simulink model "DYN_02x"  (R2021a)
settings: Solver=FixedStepAuto  StartTime=0.0  StopTime=10  FixedStep=0.01  RelTol=1e-3
(part 14 of 14)

== matlab function DYN_02x/Data ==
  data: m output; L output; Pic output; I output
function [m,L,Pic,I] = DATA_6DOF()
a1=0.75; a2=2.70; a3=0.90; d1=3.35; d4=2.95; d7=0.80;
m0 = 7.2407; m1 = 5.6511; m2 = 4.6061; m3 = 4.2963; m4 = 1.9151; m5 = 0.3399; m6 = 0.0714;
m = [m1 m2 m3 m4 m5 m6];
L = [a1 a2 a3 d1 d4 d7];
Pic = zeros(6,3);
I = zeros(6,6);
